simulink model "Sanepa_overall_model0x2810x29copy"  (R2022a)
settings: Solver=VariableStepAuto  StartTime=0.0  StopTime=1  RelTol=1e-3
undefined symbols (not defined in the file): D11, Delta
libraries: spsSeriesRLCLoadLib x54, spsLoadFlowBusLib x45, spsThreePhaseTransformerTwoWindingsLib x23, spsThreePhasePISectionLineLib x18, spsRMSLib x8, spsThreePhaseParallelRLCLoadLib x6, spsCurrentMeasurementLib x3, spsVoltageMeasurementLib x3, spsThreePhaseVIMeasurementLib x2, spsThreePhaseSeriesRLCBranchLib x2, spsGroundLib x1, spspowerguiLib x1
settings Model: Creator=Isha Tiwari  LastModifiedBy=neshan
settings SolverCC: AlgebraicLoopSolver=TrustRegion
settings DataIOCC: SaveOutput=off  ReturnWorkspaceOutputs=off
settings DebuggingCC: SFMachineParentedDataDiag=warning
settings ModelReferenceCC: EnableRefExpFcnMdlSchedulingChecks=off
settings RTWCC: Description=Generic Real-Time Target

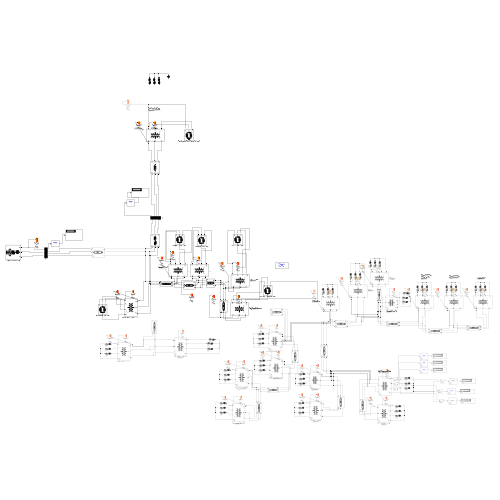
[thumbnail: Simulink's stored preview of the top-level diagram]
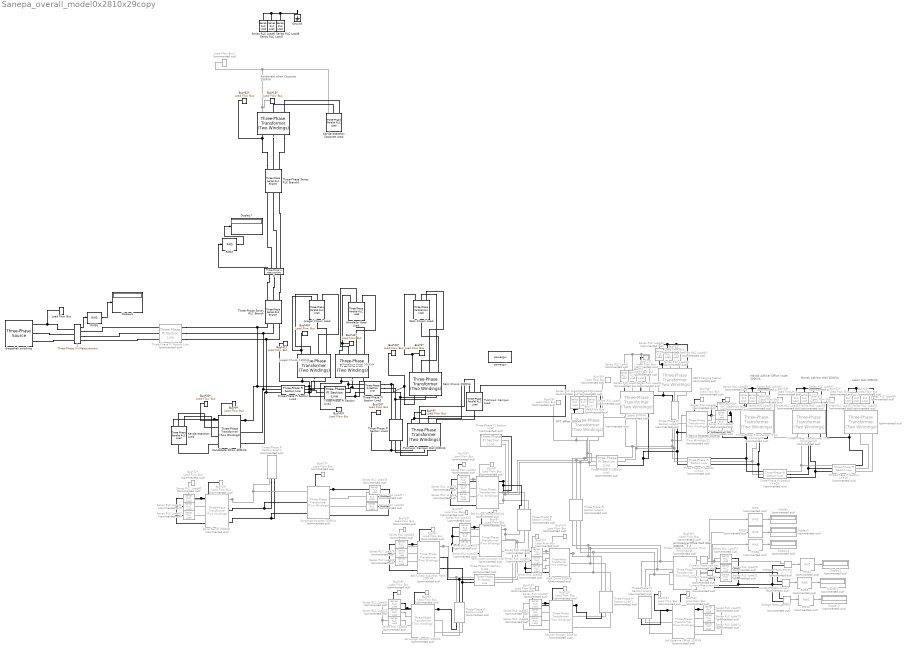
== system Sanepa_overall_model0x2810x29copy ==
  note: Norvic Hospital
      | 200KVA
  note: NTC office
      | 200KVA
  note: Manab Adhikar
      | Office inside
      | 200KVA
  note: Labim Mall
      | 200KVA
  note: Jal Utpanna Office
      | Wall Side 200KVA
  note: Manab Adhikar
      | Wall 200KVA
  note: Jwagal Chwok
      | 100KVA
  note: Himalaya Hotel
      | 300KVA
  note: Kandevata sthan
      | Opposite 250KVA
  . : spsThreePhaseTransformerTwoWindingsLib/Three-Phase Transformer (Two Windings)  Winding1Connection=Yg  Winding2Connection=Yg  CoreType=Three-limb core (core-type)  SetSaturation=off  Hysteresis=off  DataFile='hysteresis'  SetInitialFlux=off  Measurements=None  UNITS=pu  NominalPower=[ 500000 , 50 ]  Winding1=[11e3 , 0.002 , 0.08 ]  Winding2=[ 0.23e3 , 0.002 , 0.08 ]  Rm=500  Lm=500  L0=0.5  Saturation=[ 0,0 ; 0.0024,1.2 ; 1.0,1.52 ]  InitialFluxes=[ 0.8 , -0.8 , 0.7 ]  BreakLoop=off  DiscreteSolver=Trapezoidal iterative  DataType=off  TransfoNumber=1
  .. : spsThreePhaseTransformerTwoWindingsLib/Three-Phase Transformer (Two Windings)  Commented=on  Winding1Connection=Delta (D11)  Winding2Connection=Yn  CoreType=Three single-phase transformers  SetSaturation=off  Hysteresis=off  DataFile='hysteresis'  SetInitialFlux=off  Measurements=None  UNITS=pu  NominalPower=[ 200000 , 50 ]  Winding1=[ 11e3 , 0.002 , 0.08 ]  Winding2=[ 0.23e3 , 0.002 , 0.08 ]  Rm=500  Lm=500  L0=0.5  Saturation=[ 0,0 ; 0.0024,1.2 ; 1.0,1.52 ]  InitialFluxes=[ 0.8 , -0.8 , 0.7 ]  BreakLoop=off  DiscreteSolver=Trapezoidal iterative  DataType=off  TransfoNumber=1
  ... : spsThreePhaseTransformerTwoWindingsLib/Three-Phase Transformer (Two Windings)  Commented=on  Winding1Connection=Delta (D11)  Winding2Connection=Yn  CoreType=Three single-phase transformers  SetSaturation=off  Hysteresis=off  DataFile='hysteresis'  SetInitialFlux=off  Measurements=None  UNITS=pu  NominalPower=[ 200000 , 50 ]  Winding1=[11e3 , 0.002 , 0.08 ]  Winding2=[ 0.23e3 , 0.002 , 0.08 ]  Rm=500  Lm=500  L0=0.5  Saturation=[ 0,0 ; 0.0024,1.2 ; 1.0,1.52 ]  InitialFluxes=[ 0.8 , -0.8 , 0.7 ]  BreakLoop=off  DiscreteSolver=Trapezoidal iterative  DataType=off  TransfoNumber=1
  0 : spsThreePhaseVIMeasurementLib/Three-Phase V-I Measurement  VoltageMeasurement=phase-to-ground  SetLabelV=off  LabelV=V0  Vpu=on  VpuLL=off  CurrentMeasurement=no  SetLabelI=on  LabelI=I634  Ipu=off  Pbase=100e6  Vbase=11000  OutputType=Magnitude  PhasorSimulation=off  PSBequivalent=0
  1 : spsThreePhaseVIMeasurementLib/Three-Phase V-I Measurement  VoltageMeasurement=phase-to-ground  SetLabelV=off  LabelV=V0  Vpu=on  VpuLL=off  CurrentMeasurement=no  SetLabelI=on  LabelI=I634  Ipu=off  Pbase=100e6  Vbase=11000  OutputType=Magnitude  PhasorSimulation=off  PSBequivalent=0
  Bakhundol Carwash 200KVA : spsThreePhaseTransformerTwoWindingsLib/Three-Phase Transformer (Two Windings)  Commented=on  Winding1Connection=Delta (D11)  Winding2Connection=Yn  CoreType=Three single-phase transformers  SetSaturation=off  Hysteresis=off  DataFile='hysteresis'  SetInitialFlux=off  Measurements=None  UNITS=pu  NominalPower=[ 200000 , 50 ]  Winding1=[ 11e3 , 0.002 , 0.08 ]  Winding2=[ 0.23e3 , 0.002 , 0.08 ]  Rm=500  Lm=500  L0=0.5  Saturation=[ 0,0 ; 0.0024,1.2 ; 1.0,1.52 ]  InitialFluxes=[ 0.8 , -0.8 , 0.7 ]  BreakLoop=off  DiscreteSolver=Trapezoidal iterative  DataType=off  TransfoNumber=1
  Bakhundol Kutumba Hotel 200KVA : spsThreePhaseTransformerTwoWindingsLib/Three-Phase Transformer (Two Windings)  Commented=on  Winding1Connection=Delta (D11)  Winding2Connection=Yn  CoreType=Three single-phase transformers  SetSaturation=off  Hysteresis=off  DataFile='hysteresis'  SetInitialFlux=off  Measurements=None  UNITS=pu  NominalPower=[ 200000 , 50 ]  Winding1=[ 11e3 , 0.002 , 0.08 ]  Winding2=[ 0.23e3 , 0.002 , 0.08 ]  Rm=500  Lm=500  L0=0.5  Saturation=[ 0,0 ; 0.0024,1.2 ; 1.0,1.52 ]  InitialFluxes=[ 0.8 , -0.8 , 0.7 ]  BreakLoop=off  DiscreteSolver=Trapezoidal iterative  DataType=off  TransfoNumber=1
  Bakhundol Mode 300KVA : spsThreePhaseTransformerTwoWindingsLib/Three-Phase Transformer (Two Windings)  Commented=on  Winding1Connection=Delta (D11)  Winding2Connection=Yn  CoreType=Three single-phase transformers  SetSaturation=off  Hysteresis=off  DataFile='hysteresis'  SetInitialFlux=off  Measurements=None  UNITS=pu  NominalPower=[ 300000 , 50 ]  Winding1=[ 11e3 , 0.002 , 0.08 ]  Winding2=[ 0.23e3 , 0.002 , 0.08 ]  Rm=500  Lm=500  L0=0.5  Saturation=[ 0,0 ; 0.0024,1.2 ; 1.0,1.52 ]  InitialFluxes=[ 0.8 , -0.8 , 0.7 ]  BreakLoop=off  DiscreteSolver=Trapezoidal iterative  DataType=off  TransfoNumber=1
  Bima Samiti 200KVA : spsThreePhaseTransformerTwoWindingsLib/Three-Phase Transformer (Two Windings)  Commented=on  Winding1Connection=Delta (D11)  Winding2Connection=Yn  CoreType=Three single-phase transformers  SetSaturation=off  Hysteresis=off  DataFile='hysteresis'  SetInitialFlux=off  Measurements=None  UNITS=pu  NominalPower=[ 200000 , 50 ]  Winding1=[ 11e3 , 0.002 , 0.08 ]  Winding2=[ 0.23e3 , 0.002 , 0.08 ]  Rm=500  Lm=500  L0=0.5  Saturation=[ 0,0 ; 0.0024,1.2 ; 1.0,1.52 ]  InitialFluxes=[ 0.8 , -0.8 , 0.7 ]  BreakLoop=off  DiscreteSolver=Trapezoidal iterative  DataType=off  TransfoNumber=1
  Bus*1* : spsLoadFlowBusLib/Load Flow Bus  Commented=on  LConnTagsString=a  Phases=single  Connectors=on one side  ID=Bus*1*  Vbase=400  Vref=1  Vangle=0  VLF=1  VLFb=1  VLFc=1  angleLF=0  angleLFb=0  angleLFc=0
      settings: SourceProductBaseCode=PS
  Bus*10* : spsLoadFlowBusLib/Load Flow Bus  Commented=on  LConnTagsString=a  Phases=single  Connectors=on one side  ID=Bus*10*  Vbase=230  Vref=1  Vangle=0  VLF=1  VLFb=1  VLFc=1  angleLF=0  angleLFb=0  angleLFc=0
      settings: SourceProductBaseCode=PS
  Bus*11* : spsLoadFlowBusLib/Load Flow Bus  Commented=on  LConnTagsString=a  Phases=single  Connectors=on one side  ID=Bus*11*  Vbase=230  Vref=1  Vangle=0  VLF=1  VLFb=1  VLFc=1  angleLF=0  angleLFb=0  angleLFc=0
      settings: SourceProductBaseCode=PS
  Bus*12* : spsLoadFlowBusLib/Load Flow Bus  Commented=on  LConnTagsString=a  Phases=single  Connectors=on one side  ID=Bus*12*  Vbase=230  Vref=1  Vangle=0  VLF=1  VLFb=1  VLFc=1  angleLF=0  angleLFb=0  angleLFc=0
      settings: SourceProductBaseCode=PS
  Bus*13* : spsLoadFlowBusLib/Load Flow Bus  LConnTagsString=a  Phases=single  Connectors=on one side  ID=Bus*13*  Vbase=230  Vref=1  Vangle=0  VLF=0.9989  VLFb=1  VLFc=1  angleLF=-0.1488  angleLFb=0  angleLFc=0
      settings: SourceProductBaseCode=PS
  Bus*14* : spsLoadFlowBusLib/Load Flow Bus  Commented=on  LConnTagsString=a  Phases=single  Connectors=on one side  ID=Bus*14*  Vbase=230  Vref=1  Vangle=0  VLF=1  VLFb=1  VLFc=1  angleLF=0  angleLFb=0  angleLFc=0
      settings: SourceProductBaseCode=PS
  Bus*15* : spsLoadFlowBusLib/Load Flow Bus  Commented=on  LConnTagsString=a  Phases=single  Connectors=on one side  ID=Bus*15*  Vbase=230  Vref=1  Vangle=0  VLF=1  VLFb=1  VLFc=1  angleLF=0  angleLFb=0  angleLFc=0
      settings: SourceProductBaseCode=PS
  Bus*16* : spsLoadFlowBusLib/Load Flow Bus  Commented=on  LConnTagsString=a  Phases=single  Connectors=on one side  ID=Bus*16*  Vbase=230  Vref=1  Vangle=0  VLF=1  VLFb=1  VLFc=1  angleLF=0  angleLFb=0  angleLFc=0
      settings: SourceProductBaseCode=PS
  Bus*17* : spsLoadFlowBusLib/Load Flow Bus  Commented=on  LConnTagsString=a  Phases=single  Connectors=on one side  ID=Bus*17*  Vbase=230  Vref=1  Vangle=0  VLF=1  VLFb=1  VLFc=1  angleLF=0  angleLFb=0  angleLFc=0
      settings: SourceProductBaseCode=PS
  Bus*18* : spsLoadFlowBusLib/Load Flow Bus  Commented=on  LConnTagsString=a  Phases=single  Connectors=on one side  ID=Bus*18*  Vbase=11000  Vref=1  Vangle=0  VLF=1  VLFb=1  VLFc=1  angleLF=0  angleLFb=0  angleLFc=0
      settings: SourceProductBaseCode=PS
  Bus*19* : spsLoadFlowBusLib/Load Flow Bus  Commented=on  LConnTagsString=a  Phases=single  Connectors=on one side  ID=Bus*19*  Vbase=11000  Vref=1  Vangle=0  VLF=1  VLFb=1  VLFc=1  angleLF=0  angleLFb=0  angleLFc=0
      settings: SourceProductBaseCode=PS
  Bus*2* : spsLoadFlowBusLib/Load Flow Bus  LConnTagsString=a  Phases=single  Connectors=on one side  ID=Bus*2*  Vbase=230  Vref=1  Vangle=0  VLF=1  VLFb=1  VLFc=1  angleLF=0  angleLFb=0  angleLFc=0
      settings: SourceProductBaseCode=PS
  Bus*20* : spsLoadFlowBusLib/Load Flow Bus  Commented=on  LConnTagsString=a  Phases=single  Connectors=on one side  ID=Bus*20*  Vbase=11000  Vref=1  Vangle=0  VLF=1  VLFb=1  VLFc=1  angleLF=0  angleLFb=0  angleLFc=0
      settings: SourceProductBaseCode=PS
  Bus*21* : spsLoadFlowBusLib/Load Flow Bus  Commented=on  LConnTagsString=a  Phases=single  Connectors=on one side  ID=Bus*21*  Vbase=11000  Vref=1  Vangle=0  VLF=1  VLFb=1  VLFc=1  angleLF=0  angleLFb=0  angleLFc=0
      settings: SourceProductBaseCode=PS
  Bus*22* : spsLoadFlowBusLib/Load Flow Bus  Commented=on  LConnTagsString=a  Phases=single  Connectors=on one side  ID=Bus*22*  Vbase=11000  Vref=1  Vangle=0  VLF=1  VLFb=1  VLFc=1  angleLF=0  angleLFb=0  angleLFc=0
      settings: SourceProductBaseCode=PS
  Bus*23* : spsLoadFlowBusLib/Load Flow Bus  LConnTagsString=a  Phases=single  Connectors=on one side  ID=Bus*23*  Vbase=11000  Vref=1  Vangle=0  VLF=1  VLFb=1  VLFc=1  angleLF=0  angleLFb=0  angleLFc=0
      settings: SourceProductBaseCode=PS
  Bus*24* : spsLoadFlowBusLib/Load Flow Bus  Commented=on  LConnTagsString=a  Phases=single  Connectors=on one side  ID=Bus*24*  Vbase=11000  Vref=1  Vangle=0  VLF=1  VLFb=1  VLFc=1  angleLF=0  angleLFb=0  angleLFc=0
      settings: SourceProductBaseCode=PS
  Bus*25* : spsLoadFlowBusLib/Load Flow Bus  Commented=on  LConnTagsString=a  Phases=single  Connectors=on one side  ID=Bus*25*  Vbase=11000  Vref=1  Vangle=0  VLF=1  VLFb=1  VLFc=1  angleLF=0  angleLFb=0  angleLFc=0
      settings: SourceProductBaseCode=PS
  Bus*26* : spsLoadFlowBusLib/Load Flow Bus  LConnTagsString=a  Phases=single  Connectors=on one side  ID=Bus*26*  Vbase=11000  Vref=1  Vangle=0  VLF=1  VLFb=1  VLFc=1  angleLF=0  angleLFb=0  angleLFc=0
      settings: SourceProductBaseCode=PS
  Bus*27* : spsLoadFlowBusLib/Load Flow Bus  Commented=on  LConnTagsString=a  Phases=single  Connectors=on one side  ID=Bus*27*  Vbase=11000  Vref=1  Vangle=0  VLF=1  VLFb=1  VLFc=1  angleLF=0  angleLFb=0  angleLFc=0
      settings: SourceProductBaseCode=PS
  Bus*28* : spsLoadFlowBusLib/Load Flow Bus  Commented=on  LConnTagsString=a  Phases=single  Connectors=on one side  ID=Bus*28*  Vbase=11000  Vref=1  Vangle=0  VLF=1  VLFb=1  VLFc=1  angleLF=0  angleLFb=0  angleLFc=0
      settings: SourceProductBaseCode=PS
  Bus*29* : spsLoadFlowBusLib/Load Flow Bus  Commented=on  LConnTagsString=a  Phases=single  Connectors=on one side  ID=Bus*29*  Vbase=11000  Vref=1  Vangle=0  VLF=1  VLFb=1  VLFc=1  angleLF=0  angleLFb=0  angleLFc=0
      settings: SourceProductBaseCode=PS
  Bus*3* : spsLoadFlowBusLib/Load Flow Bus  LConnTagsString=a  Phases=single  Connectors=on one side  ID=Bus*3*  Vbase=230  Vref=1  Vangle=0  VLF=1  VLFb=1  VLFc=1  angleLF=0  angleLFb=0  angleLFc=0
      settings: SourceProductBaseCode=PS
  Bus*30* : spsLoadFlowBusLib/Load Flow Bus  LConnTagsString=a  Phases=single  Connectors=on one side  ID=Bus*30*  Vbase=11000  Vref=1  Vangle=0  VLF=1  VLFb=1  VLFc=1  angleLF=0  angleLFb=0  angleLFc=0
      settings: SourceProductBaseCode=PS
  Bus*31* : spsLoadFlowBusLib/Load Flow Bus  LConnTagsString=a  Phases=single  Connectors=on one side  ID=Bus*31*  Vbase=11000  Vref=1  Vangle=0  VLF=0.9999  VLFb=1  VLFc=1  angleLF=-0.004876  angleLFb=0  angleLFc=0
      settings: SourceProductBaseCode=PS
  Bus*32* : spsLoadFlowBusLib/Load Flow Bus  Commented=on  LConnTagsString=a  Phases=single  Connectors=on one side  ID=Bus*32*  Vbase=230  Vref=1  Vangle=0  VLF=1  VLFb=1  VLFc=1  angleLF=0  angleLFb=0  angleLFc=0
      settings: SourceProductBaseCode=PS
  Bus*33* : spsLoadFlowBusLib/Load Flow Bus  Commented=on  LConnTagsString=a  Phases=single  Connectors=on one side  ID=Bus*33*  Vbase=11000  Vref=1  Vangle=0  VLF=1  VLFb=1  VLFc=1  angleLF=0  angleLFb=0  angleLFc=0
      settings: SourceProductBaseCode=PS
  Bus*34* : spsLoadFlowBusLib/Load Flow Bus  Commented=on  LConnTagsString=a  Phases=single  Connectors=on one side  ID=Bus*34*  Vbase=230  Vref=1  Vangle=0  VLF=1  VLFb=1  VLFc=1  angleLF=0  angleLFb=0  angleLFc=0
      settings: SourceProductBaseCode=PS
  Bus*35* : spsLoadFlowBusLib/Load Flow Bus  Commented=on  LConnTagsString=a  Phases=single  Connectors=on one side  ID=Bus*35*  Vbase=11000  Vref=1  Vangle=0  VLF=1  VLFb=1  VLFc=1  angleLF=0  angleLFb=0  angleLFc=0
      settings: SourceProductBaseCode=PS
  Bus*36* : spsLoadFlowBusLib/Load Flow Bus  Commented=on  LConnTagsString=a  Phases=single  Connectors=on one side  ID=Bus*36*  Vbase=230  Vref=1  Vangle=0  VLF=1  VLFb=1  VLFc=1  angleLF=0  angleLFb=0  angleLFc=0
      settings: SourceProductBaseCode=PS
  Bus*37* : spsLoadFlowBusLib/Load Flow Bus  Commented=on  LConnTagsString=a  Phases=single  Connectors=on one side  ID=Bus*37*  Vbase=11000  Vref=1  Vangle=0  VLF=1  VLFb=1  VLFc=1  angleLF=0  angleLFb=0  angleLFc=0
      settings: SourceProductBaseCode=PS
  Bus*38* : spsLoadFlowBusLib/Load Flow Bus  Commented=on  LConnTagsString=a  Phases=single  Connectors=on one side  ID=Bus*38*  Vbase=230  Vref=1  Vangle=0  VLF=1  VLFb=1  VLFc=1  angleLF=0  angleLFb=0  angleLFc=0
      settings: SourceProductBaseCode=PS
  Bus*39* : spsLoadFlowBusLib/Load Flow Bus  Commented=on  LConnTagsString=a  Phases=single  Connectors=on one side  ID=Bus*39*  Vbase=11000  Vref=1  Vangle=0  VLF=1  VLFb=1  VLFc=1  angleLF=0  angleLFb=0  angleLFc=0
      settings: SourceProductBaseCode=PS
  Bus*4* : spsLoadFlowBusLib/Load Flow Bus  Commented=on  LConnTagsString=a  Phases=single  Connectors=on one side  ID=Bus*4*  Vbase=230  Vref=1  Vangle=0  VLF=1  VLFb=1  VLFc=1  angleLF=0  angleLFb=0  angleLFc=0
      settings: SourceProductBaseCode=PS
  Bus*40* : spsLoadFlowBusLib/Load Flow Bus  LConnTagsString=a  Phases=single  Connectors=on one side  ID=Bus*40*  Vbase=230  Vref=1  Vangle=0  VLF=1  VLFb=1  VLFc=1  angleLF=0  angleLFb=0  angleLFc=0
      settings: SourceProductBaseCode=PS
  Bus*41* : spsLoadFlowBusLib/Load Flow Bus  LConnTagsString=a  Phases=single  Connectors=on one side  ID=Bus*41*  Vbase=11000  Vref=1  Vangle=0  VLF=1  VLFb=1  VLFc=1  angleLF=0  angleLFb=0  angleLFc=0
      settings: SourceProductBaseCode=PS
  Bus*42* : spsLoadFlowBusLib/Load Flow Bus  LConnTagsString=a  Phases=single  Connectors=on one side  ID=Bus*42*  Vbase=230  Vref=1  Vangle=0  VLF=1  VLFb=1  VLFc=1  angleLF=0  angleLFb=0  angleLFc=0
      settings: SourceProductBaseCode=PS
  Bus*43* : spsLoadFlowBusLib/Load Flow Bus  LConnTagsString=a  Phases=single  Connectors=on one side  ID=Bus*43*  Vbase=11000  Vref=1  Vangle=0  VLF=1  VLFb=1  VLFc=1  angleLF=0  angleLFb=0  angleLFc=0
      settings: SourceProductBaseCode=PS
  Bus*5* : spsLoadFlowBusLib/Load Flow Bus  Commented=on  LConnTagsString=a  Phases=single  Connectors=on one side  ID=Bus*5*  Vbase=230  Vref=1  Vangle=0  VLF=1  VLFb=1  VLFc=1  angleLF=0  angleLFb=0  angleLFc=0
      settings: SourceProductBaseCode=PS
  Bus*6* : spsLoadFlowBusLib/Load Flow Bus  Commented=on  LConnTagsString=a  Phases=single  Connectors=on one side  ID=Bus*6*  Vbase=230  Vref=1  Vangle=0  VLF=1  VLFb=1  VLFc=1  angleLF=0  angleLFb=0  angleLFc=0
      settings: SourceProductBaseCode=PS
  Bus*7* : spsLoadFlowBusLib/Load Flow Bus  Commented=on  LConnTagsString=a  Phases=single  Connectors=on one side  ID=Bus*7*  Vbase=230  Vref=1  Vangle=0  VLF=1  VLFb=1  VLFc=1  angleLF=0  angleLFb=0  angleLFc=0
      settings: SourceProductBaseCode=PS
  Bus*8* : spsLoadFlowBusLib/Load Flow Bus  Commented=on  LConnTagsString=a  Phases=single  Connectors=on one side  ID=Bus*8*  Vbase=230  Vref=1  Vangle=0  VLF=1  VLFb=1  VLFc=1  angleLF=0  angleLFb=0  angleLFc=0
      settings: SourceProductBaseCode=PS
  Bus*9* : spsLoadFlowBusLib/Load Flow Bus  LConnTagsString=a  Phases=single  Connectors=on one side  ID=Bus*9*  Vbase=230  Vref=1  Vangle=0  VLF=1  VLFb=1  VLFc=1  angleLF=0  angleLFb=0  angleLFc=0
      settings: SourceProductBaseCode=PS
  Current Measurement : spsCurrentMeasurementLib/Current Measurement  Commented=on  PhasorSimulation=off  OutputType=Complex  PSBequivalent=0
  Current Measurement3 : spsCurrentMeasurementLib/Current Measurement  Commented=on  PhasorSimulation=off  OutputType=Complex  PSBequivalent=0
  Current Measurement4 : spsCurrentMeasurementLib/Current Measurement  Commented=on  PhasorSimulation=off  OutputType=Complex  PSBequivalent=0
  Display{,1..5} (6 alike) : Display  Commented=on
  Display6 : Display
  Display7 : Display
  Ground : spsGroundLib/Ground  LConnTagsString=a
  HImalaya Hotel Load : spsThreePhaseParallelRLCLoadLib/Three-Phase Parallel RLC Load  LConnTagsString=A|B|C  RConnTagsString=N  Configuration=Y (neutral)  NominalVoltage=230  Vabc=[1e3 1e3 1e3]  Vabcp=[1e3 1e3 1e3]  NominalFrequency=50  UnbalancedPower=off  ActivePower=29497.5  InductivePower=9695.359  CapacitivePower=0  Pabc=[22287 23379.5 18572.5]  QLabc=[7325.383 7684.47 6104.48]  QCabc=[0 0 0]  Pabcp=[10e3 9e3 11e3]  QLabcp=[100 90 110]  QCabcp=[100 90 110]  Measurements=None  LoadType=constant PQ
  High Court 200KVA : spsThreePhaseTransformerTwoWindingsLib/Three-Phase Transformer (Two Windings)  Commented=on  Winding1Connection=Delta (D11)  Winding2Connection=Yn  CoreType=Three single-phase transformers  SetSaturation=off  Hysteresis=off  DataFile='hysteresis'  SetInitialFlux=off  Measurements=None  UNITS=pu  NominalPower=[ 200000 , 50 ]  Winding1=[ 11e3 , 0.002 , 0.08 ]  Winding2=[ 0.23e3 , 0.002 , 0.08 ]  Rm=500  Lm=500  L0=0.5  Saturation=[ 0,0 ; 0.0024,1.2 ; 1.0,1.52 ]  InitialFluxes=[ 0.8 , -0.8 , 0.7 ]  BreakLoop=off  DiscreteSolver=Trapezoidal iterative  DataType=off  TransfoNumber=1
  Jall Utpanna Office 100KVA : spsThreePhaseTransformerTwoWindingsLib/Three-Phase Transformer (Two Windings)  Commented=on  Winding1Connection=Delta (D11)  Winding2Connection=Yn  CoreType=Three single-phase transformers  SetSaturation=off  Hysteresis=off  DataFile='hysteresis'  SetInitialFlux=off  Measurements=None  UNITS=pu  NominalPower=[ 100000 , 50 ]  Winding1=[ 11e3 , 0.002 , 0.08 ]  Winding2=[ 0.23e3 , 0.002 , 0.08 ]  Rm=500  Lm=500  L0=0.5  Saturation=[ 0,0 ; 0.0024,1.2 ; 1.0,1.52 ]  InitialFluxes=[ 0.8 , -0.8 , 0.7 ]  BreakLoop=off  DiscreteSolver=Trapezoidal iterative  DataType=off  TransfoNumber=1
  Jwagal Chowk Load : spsThreePhaseParallelRLCLoadLib/Three-Phase Parallel RLC Load  LConnTagsString=A|B|C  RConnTagsString=N  Configuration=Y (neutral)  NominalVoltage=230  Vabc=[1e3 1e3 1e3]  Vabcp=[1e3 1e3 1e3]  NominalFrequency=50  UnbalancedPower=off  ActivePower=21850  InductivePower=7181.748  CapacitivePower=0  Pabc=[22287 23379.5 18572.5]  QLabc=[7325.383 7684.47 6104.48]  QCabc=[0 0 0]  Pabcp=[10e3 9e3 11e3]  QLabcp=[100 90 110]  QCabcp=[100 90 110]  Measurements=None  LoadType=constant PQ
  Kandebata Sthan 300KVA : spsThreePhaseTransformerTwoWindingsLib/Three-Phase Transformer (Two Windings)  Winding1Connection=Delta (D11)  Winding2Connection=Yn  CoreType=Three single-phase transformers  SetSaturation=off  Hysteresis=off  DataFile='hysteresis'  SetInitialFlux=off  Measurements=None  UNITS=pu  NominalPower=[ 300000 , 50 ]  Winding1=[ 11e3 , 0.002 , 0.08 ]  Winding2=[ 0.23e3 , 0.002 , 0.08 ]  Rm=500  Lm=500  L0=0.5  Saturation=[ 0,0 ; 0.0024,1.2 ; 1.0,1.52 ]  InitialFluxes=[ 0.8 , -0.8 , 0.7 ]  BreakLoop=off  DiscreteSolver=Trapezoidal iterative  DataType=off  TransfoNumber=1
  Kandevatasthan Load : spsThreePhaseParallelRLCLoadLib/Three-Phase Parallel RLC Load  LConnTagsString=A|B|C  RConnTagsString=N  Configuration=Y (neutral)  NominalVoltage=230  Vabc=[1e3 1e3 1e3]  Vabcp=[1e3 1e3 1e3]  NominalFrequency=50  UnbalancedPower=off  ActivePower=68827.5  InductivePower=22622.506  CapacitivePower=0  Pabc=[22287 23379.5 18572.5]  QLabc=[7325.383 7684.47 6104.48]  QCabc=[0 0 0]  Pabcp=[10e3 9e3 11e3]  QLabcp=[100 90 110]  QCabcp=[100 90 110]  Measurements=None  LoadType=constant PQ
  Kandevatasthan Opposite Load : spsThreePhaseParallelRLCLoadLib/Three-Phase Parallel RLC Load  LConnTagsString=A|B|C  Configuration=Y (grounded)  NominalVoltage=230  Vabc=[1e3 1e3 1e3]  Vabcp=[1e3 1e3 1e3]  NominalFrequency=50  UnbalancedPower=off  ActivePower=64239  InductivePower=21114.33  CapacitivePower=0  Pabc=[22287 23379.5 18572.5]  QLabc=[7325.383 7684.47 6104.48]  QCabc=[0 0 0]  Pabcp=[10e3 9e3 11e3]  QLabcp=[100 90 110]  QCabcp=[100 90 110]  Measurements=None  LoadType=constant PQ
  Load Flow Bus : spsLoadFlowBusLib/Load Flow Bus  LConnTagsString=a  Phases=single  Connectors=on one side  ID=BUS_1  Vbase=11e3  Vref=1  Vangle=0  VLF=1  VLFb=1  VLFc=1  angleLF=0  angleLFb=0  angleLFc=0
      settings: SourceProductBaseCode=PS
  Load Flow Bus1 : spsLoadFlowBusLib/Load Flow Bus  Commented=on  LConnTagsString=a  Phases=single  Connectors=on one side  ID=BUS_2  Vbase=11e3  Vref=1  Vangle=0  VLF=1  VLFb=1  VLFc=1  angleLF=0  angleLFb=0  angleLFc=0
      settings: SourceProductBaseCode=PS
  NEA Charging Station : spsThreePhaseTransformerTwoWindingsLib/Three-Phase Transformer (Two Windings)  Commented=on  Winding1Connection=Delta (D11)  Winding2Connection=Yn  CoreType=Three single-phase transformers  SetSaturation=off  Hysteresis=off  DataFile='hysteresis'  SetInitialFlux=off  Measurements=None  UNITS=pu  NominalPower=[ 200000 , 50 ]  Winding1=[ 11e3 , 0.002 , 0.08 ]  Winding2=[ 0.23e3 , 0.002 , 0.08 ]  Rm=500  Lm=500  L0=0.5  Saturation=[ 0,0 ; 0.0024,1.2 ; 1.0,1.52 ]  InitialFluxes=[ 0.8 , -0.8 , 0.7 ]  BreakLoop=off  DiscreteSolver=Trapezoidal iterative  DataType=off  TransfoNumber=1
  Pariwar Niyojan 100KVA : spsThreePhaseTransformerTwoWindingsLib/Three-Phase Transformer (Two Windings)  Commented=on  Winding1Connection=Delta (D11)  Winding2Connection=Yn  CoreType=Three single-phase transformers  SetSaturation=off  Hysteresis=off  DataFile='hysteresis'  SetInitialFlux=off  Measurements=None  UNITS=pu  NominalPower=[ 100000 , 50 ]  Winding1=[ 11e3 , 0.002 , 0.08 ]  Winding2=[ 0.23e3 , 0.002 , 0.08 ]  Rm=500  Lm=500  L0=0.5  Saturation=[ 0,0 ; 0.0024,1.2 ; 1.0,1.52 ]  InitialFluxes=[ 0.8 , -0.8 , 0.7 ]  BreakLoop=off  DiscreteSolver=Trapezoidal iterative  DataType=off  TransfoNumber=1
  Pulchowk Campus Load : spsThreePhaseParallelRLCLoadLib/Three-Phase Parallel RLC Load  LConnTagsString=A|B|C  RConnTagsString=N  Configuration=Y (neutral)  NominalVoltage=230  Vabc=[1e3 1e3 1e3]  Vabcp=[1e3 1e3 1e3]  NominalFrequency=50  UnbalancedPower=off  ActivePower=38019.33  InductivePower=12496.241  CapacitivePower=0  Pabc=[22287 23379.5 18572.5]  QLabc=[7325.383 7684.47 6104.48]  QCabc=[0 0 0]  Pabcp=[10e3 9e3 11e3]  QLabcp=[100 90 110]  QCabcp=[100 90 110]  Measurements=None  LoadType=constant PQ
  Pulchwok Campus Wall 200KVA : spsThreePhaseTransformerTwoWindingsLib/Three-Phase Transformer (Two Windings)  Winding1Connection=Delta (D11)  Winding2Connection=Yn  CoreType=Three single-phase transformers  SetSaturation=off  Hysteresis=off  DataFile='hysteresis'  SetInitialFlux=off  Measurements=None  UNITS=pu  NominalPower=[ 100000 , 50 ]  Winding1=[ 11e3 , 0.002 , 0.08 ]  Winding2=[ 0.23e3 , 0.002 , 0.08 ]  Rm=500  Lm=500  L0=0.5  Saturation=[ 0,0 ; 0.0024,1.2 ; 1.0,1.52 ]  InitialFluxes=[ 0.8 , -0.8 , 0.7 ]  BreakLoop=off  DiscreteSolver=Trapezoidal iterative  DataType=off  TransfoNumber=1
  RMS{,1..5} (6 alike) : spsRMSLib/RMS  Commented=on  TrueRMS=on  Freq=50  RMSInit=0  Ts=0
  RMS6 : spsRMSLib/RMS  TrueRMS=on  Freq=60  RMSInit=120  Ts=0
  RMS7 : spsRMSLib/RMS  TrueRMS=on  Freq=60  RMSInit=0  Ts=0
  Sajha 500KVA : spsThreePhaseTransformerTwoWindingsLib/Three-Phase Transformer (Two Windings)  Commented=on  Winding1Connection=Delta (D11)  Winding2Connection=Yn  CoreType=Three single-phase transformers  SetSaturation=off  Hysteresis=off  DataFile='hysteresis'  SetInitialFlux=off  Measurements=None  UNITS=pu  NominalPower=[ 500000 , 50 ]  Winding1=[ 11e3 , 0.002 , 0.08 ]  Winding2=[ 0.40e3 , 0.002 , 0.08 ]  Rm=500  Lm=500  L0=0.5  Saturation=[ 0,0 ; 0.0024,1.2 ; 1.0,1.52 ]  InitialFluxes=[ 0.8 , -0.8 , 0.7 ]  BreakLoop=off  DiscreteSolver=Trapezoidal iterative  DataType=off  TransfoNumber=1
  Salik Chowk Load : spsThreePhaseParallelRLCLoadLib/Three-Phase Parallel RLC Load  LConnTagsString=A|B|C  RConnTagsString=N  Configuration=Y (neutral)  NominalVoltage=230  Vabc=[1e3 1e3 1e3]  Vabcp=[1e3 1e3 1e3]  NominalFrequency=50  UnbalancedPower=off  ActivePower=19883.5  InductivePower=6535.388  CapacitivePower=0  Pabc=[22287 23379.5 18572.5]  QLabc=[7325.383 7684.47 6104.48]  QCabc=[0 0 0]  Pabcp=[10e3 9e3 11e3]  QLabcp=[100 90 110]  QCabcp=[100 90 110]  Measurements=None  LoadType=constant PQ
  Salik Chwok 200KVA : spsThreePhaseTransformerTwoWindingsLib/Three-Phase Transformer (Two Windings)  Winding1Connection=Delta (D11)  Winding2Connection=Yn  CoreType=Three single-phase transformers  SetSaturation=off  Hysteresis=off  DataFile='hysteresis'  SetInitialFlux=off  Measurements=None  UNITS=pu  NominalPower=[ 200000 , 50 ]  Winding1=[11e3 , 0.002 , 0.08 ]  Winding2=[ 0.23e3 , 0.002 , 0.08 ]  Rm=500  Lm=500  L0=0.5  Saturation=[ 0,0 ; 0.0024,1.2 ; 1.0,1.52 ]  InitialFluxes=[ 0.8 , -0.8 , 0.7 ]  BreakLoop=off  DiscreteSolver=Trapezoidal iterative  DataType=off  TransfoNumber=1
  Sarbanga Hospital 200KVA : spsThreePhaseTransformerTwoWindingsLib/Three-Phase Transformer (Two Windings)  Commented=on  Winding1Connection=Delta (D11)  Winding2Connection=Yn  CoreType=Three single-phase transformers  SetSaturation=off  Hysteresis=off  DataFile='hysteresis'  SetInitialFlux=off  Measurements=None  UNITS=pu  NominalPower=[ 200000 , 50 ]  Winding1=[ 11e3 , 0.002 , 0.08 ]  Winding2=[ 0.23e3 , 0.002 , 0.08 ]  Rm=500  Lm=500  L0=0.5  Saturation=[ 0,0 ; 0.0024,1.2 ; 1.0,1.52 ]  InitialFluxes=[ 0.8 , -0.8 , 0.7 ]  BreakLoop=off  DiscreteSolver=Trapezoidal iterative  DataType=off  TransfoNumber=1
  Sarwanga Hospital 300KVA : spsThreePhaseTransformerTwoWindingsLib/Three-Phase Transformer (Two Windings)  Commented=on  Winding1Connection=Delta (D11)  Winding2Connection=Yn  CoreType=Three single-phase transformers  SetSaturation=off  Hysteresis=off  DataFile='hysteresis'  SetInitialFlux=off  Measurements=None  UNITS=pu  NominalPower=[ 300000 , 50 ]  Winding1=[ 11e3 , 0.002 , 0.08 ]  Winding2=[ 0.23e3 , 0.002 , 0.08 ]  Rm=500  Lm=500  L0=0.5  Saturation=[ 0,0 ; 0.0024,1.2 ; 1.0,1.52 ]  InitialFluxes=[ 0.8 , -0.8 , 0.7 ]  BreakLoop=off  DiscreteSolver=Trapezoidal iterative  DataType=off  TransfoNumber=1
  Series RLC Load1 : spsSeriesRLCLoadLib/Series RLC Load  Commented=on  LConnTagsString=a  RConnTagsString=__new0  NominalVoltage=230  NominalFrequency=50  ActivePower=50255  InductivePower=16518.02  CapacitivePower=0  Setx0=off  InitialVoltage=0  SetiL0=off  InitialCurrent=0  Measurements=None  LoadType=constant Z
  Series RLC Load2 : spsSeriesRLCLoadLib/Series RLC Load  Commented=on  LConnTagsString=a  RConnTagsString=__new0  NominalVoltage=230  NominalFrequency=50  ActivePower=32775  InductivePower=10772.62  CapacitivePower=0  Setx0=off  InitialVoltage=0  SetiL0=off  InitialCurrent=0  Measurements=None  LoadType=constant Z
  Series RLC Load21 : spsSeriesRLCLoadLib/Series RLC Load  Commented=on  LConnTagsString=a  RConnTagsString=__new0  NominalVoltage=230  NominalFrequency=50  ActivePower=21850  InductivePower=7181.75  CapacitivePower=0  Setx0=off  InitialVoltage=0  SetiL0=off  InitialCurrent=0  Measurements=None  LoadType=constant Z
  Series RLC Load22 : spsSeriesRLCLoadLib/Series RLC Load  Commented=on  LConnTagsString=a  RConnTagsString=__new0  NominalVoltage=230  NominalFrequency=50  ActivePower=19665  InductivePower=6463.573  CapacitivePower=0  Setx0=off  InitialVoltage=0  SetiL0=off  InitialCurrent=0  Measurements=None  LoadType=constant Z
  Series RLC Load23 : spsSeriesRLCLoadLib/Series RLC Load  Commented=on  LConnTagsString=a  RConnTagsString=__new0  NominalVoltage=230  NominalFrequency=50  ActivePower=19446.5  InductivePower=6391.755  CapacitivePower=0  Setx0=off  InitialVoltage=0  SetiL0=off  InitialCurrent=0  Measurements=None  LoadType=constant Z
  Series RLC Load24 : spsSeriesRLCLoadLib/Series RLC Load  Commented=on  LConnTagsString=a  RConnTagsString=__new0  NominalVoltage=230  NominalFrequency=50  ActivePower=20539  InductivePower=6750.843  CapacitivePower=0  Setx0=off  InitialVoltage=0  SetiL0=off  InitialCurrent=0  Measurements=None  LoadType=constant Z
  Series RLC Load25 : spsSeriesRLCLoadLib/Series RLC Load  Commented=on  LConnTagsString=a  RConnTagsString=__new0  NominalVoltage=230  NominalFrequency=50  ActivePower=7647.5  InductivePower=2513.612  CapacitivePower=0  Setx0=off  InitialVoltage=0  SetiL0=off  InitialCurrent=0  Measurements=None  LoadType=constant Z
  Series RLC Load26 : spsSeriesRLCLoadLib/Series RLC Load  Commented=on  LConnTagsString=a  RConnTagsString=__new0  NominalVoltage=230  NominalFrequency=50  ActivePower=1529.5  InductivePower=502.72  CapacitivePower=0  Setx0=off  InitialVoltage=0  SetiL0=off  InitialCurrent=0  Measurements=None  LoadType=constant Z
  Series RLC Load27 : spsSeriesRLCLoadLib/Series RLC Load  Commented=on  LConnTagsString=a  RConnTagsString=__new0  NominalVoltage=230  NominalFrequency=50  ActivePower=16387.5  InductivePower=5386.311  CapacitivePower=0  Setx0=off  InitialVoltage=0  SetiL0=off  InitialCurrent=0  Measurements=None  LoadType=constant Z
  Series RLC Load28 : spsSeriesRLCLoadLib/Series RLC Load  Commented=on  LConnTagsString=a  RConnTagsString=__new0  NominalVoltage=230  NominalFrequency=50  ActivePower=5462.5  InductivePower=1795.437  CapacitivePower=0  Setx0=off  InitialVoltage=0  SetiL0=off  InitialCurrent=0  Measurements=None  LoadType=constant Z
  Series RLC Load29 : spsSeriesRLCLoadLib/Series RLC Load  Commented=on  LConnTagsString=a  RConnTagsString=__new0  NominalVoltage=230  NominalFrequency=50  ActivePower=6555  InductivePower=2154.52  CapacitivePower=0  Setx0=off  InitialVoltage=0  SetiL0=off  InitialCurrent=0  Measurements=None  LoadType=constant Z
  Series RLC Load3 : spsSeriesRLCLoadLib/Series RLC Load  Commented=on  LConnTagsString=a  RConnTagsString=__new0  NominalVoltage=230  NominalFrequency=50  ActivePower=29497.5  InductivePower=9695.359  CapacitivePower=0  Setx0=off  InitialVoltage=0  SetiL0=off  InitialCurrent=0  Measurements=None  LoadType=constant Z
  Series RLC Load30 : spsSeriesRLCLoadLib/Series RLC Load  Commented=on  LConnTagsString=a  RConnTagsString=__new0  NominalVoltage=230  NominalFrequency=50  ActivePower=3933  InductivePower=1292.715  CapacitivePower=0  Setx0=off  InitialVoltage=0  SetiL0=off  InitialCurrent=0  Measurements=None  LoadType=constant Z
  Series RLC Load31 : spsSeriesRLCLoadLib/Series RLC Load  Commented=on  LConnTagsString=a  RConnTagsString=__new0  NominalVoltage=230  NominalFrequency=50  ActivePower=19228  InductivePower=6319.938  CapacitivePower=0  Setx0=off  InitialVoltage=0  SetiL0=off  InitialCurrent=0  Measurements=None  LoadType=constant Z
  Series RLC Load32 : spsSeriesRLCLoadLib/Series RLC Load  Commented=on  LConnTagsString=a  RConnTagsString=__new0  NominalVoltage=230  NominalFrequency=50  ActivePower=16169  InductivePower=5314.493  CapacitivePower=0  Setx0=off  InitialVoltage=0  SetiL0=off  InitialCurrent=0  Measurements=None  LoadType=constant Z
  Series RLC Load33 : spsSeriesRLCLoadLib/Series RLC Load  Commented=on  LConnTagsString=a  RConnTagsString=__new0  NominalVoltage=230  NominalFrequency=50  ActivePower=15976.5  InductivePower=4955.406  CapacitivePower=0  Setx0=off  InitialVoltage=0  SetiL0=off  InitialCurrent=0  Measurements=None  LoadType=constant Z
  Series RLC Load4 : spsSeriesRLCLoadLib/Series RLC Load  Commented=on  LConnTagsString=a  RConnTagsString=__new0  NominalVoltage=230  NominalFrequency=50  ActivePower=17480  InductivePower=5745.398  CapacitivePower=0  Setx0=off  InitialVoltage=0  SetiL0=off  InitialCurrent=0  Measurements=None  LoadType=constant Z
  Series RLC Load40 : spsSeriesRLCLoadLib/Series RLC Load  Commented=on  LConnTagsString=a  RConnTagsString=__new0  NominalVoltage=230  NominalFrequency=50  ActivePower=9832.5  InductivePower=3231.786  CapacitivePower=0  Setx0=off  InitialVoltage=0  SetiL0=off  InitialCurrent=0  Measurements=None  LoadType=constant Z
  Series RLC Load41 : spsSeriesRLCLoadLib/Series RLC Load  Commented=on  LConnTagsString=a  RConnTagsString=__new0  NominalVoltage=230  NominalFrequency=50  ActivePower=9832.5  InductivePower=3231.786  CapacitivePower=0  Setx0=off  InitialVoltage=0  SetiL0=off  InitialCurrent=0  Measurements=None  LoadType=constant Z
  Series RLC Load42 : spsSeriesRLCLoadLib/Series RLC Load  Commented=on  LConnTagsString=a  RConnTagsString=__new0  NominalVoltage=230  NominalFrequency=50  ActivePower=11143.5  InductivePower=3662.691  CapacitivePower=0  Setx0=off  InitialVoltage=0  SetiL0=off  InitialCurrent=0  Measurements=None  LoadType=constant Z
  Series RLC Load{43..48,52..60} (15 alike) : spsSeriesRLCLoadLib/Series RLC Load  Commented=on  LConnTagsString=a  RConnTagsString=__new0  NominalVoltage=230  NominalFrequency=50  ActivePower=9500  InductivePower=3122.5  CapacitivePower=0  Setx0=off  InitialVoltage=0  SetiL0=off  InitialCurrent=0  Measurements=None  LoadType=constant Z
  Series RLC Load5 : spsSeriesRLCLoadLib/Series RLC Load  Commented=on  LConnTagsString=a  RConnTagsString=__new0  NominalVoltage=230  NominalFrequency=50  ActivePower=21850  InductivePower=7181.74  CapacitivePower=0  Setx0=off  InitialVoltage=0  SetiL0=off  InitialCurrent=0  Measurements=None  LoadType=constant Z
  Series RLC Load6 : spsSeriesRLCLoadLib/Series RLC Load  LConnTagsString=a  RConnTagsString=__new0  NominalVoltage=230  NominalFrequency=50  ActivePower=22287  InductivePower=7325.383  CapacitivePower=0  Setx0=off  InitialVoltage=0  SetiL0=off  InitialCurrent=0  Measurements=None  LoadType=constant Z
  Series RLC Load64 : spsSeriesRLCLoadLib/Series RLC Load  Commented=on  LConnTagsString=a  RConnTagsString=__new0  NominalVoltage=230  NominalFrequency=50  ActivePower=5899.5  InductivePower=1939.072  CapacitivePower=0  Setx0=off  InitialVoltage=0  SetiL0=off  InitialCurrent=0  Measurements=None  LoadType=constant Z
  Series RLC Load65 : spsSeriesRLCLoadLib/Series RLC Load  Commented=on  LConnTagsString=a  RConnTagsString=__new0  NominalVoltage=230  NominalFrequency=50  ActivePower=2622  InductivePower=816.8097  CapacitivePower=0  Setx0=off  InitialVoltage=0  SetiL0=off  InitialCurrent=0  Measurements=None  LoadType=constant Z
  Series RLC Load66 : spsSeriesRLCLoadLib/Series RLC Load  Commented=on  LConnTagsString=a  RConnTagsString=__new0  NominalVoltage=230  NominalFrequency=50  ActivePower=3496  InductivePower=1149.08  CapacitivePower=0  Setx0=off  InitialVoltage=0  SetiL0=off  InitialCurrent=0  Measurements=None  LoadType=constant Z
  Series RLC Load67 : spsSeriesRLCLoadLib/Series RLC Load  Commented=on  LConnTagsString=a  RConnTagsString=__new0  NominalVoltage=230  NominalFrequency=50  ActivePower=6118  InductivePower=2010.889  CapacitivePower=0  Setx0=off  InitialVoltage=0  SetiL0=off  InitialCurrent=0  Measurements=None  LoadType=constant Z
  Series RLC Load68 : spsSeriesRLCLoadLib/Series RLC Load  Commented=on  LConnTagsString=a  RConnTagsString=__new0  NominalVoltage=230  NominalFrequency=50  ActivePower=4151.5  InductivePower=1364.532  CapacitivePower=0  Setx0=off  InitialVoltage=0  SetiL0=off  InitialCurrent=0  Measurements=None  LoadType=constant Z
  Series RLC Load69 : spsSeriesRLCLoadLib/Series RLC Load  Commented=on  LConnTagsString=a  RConnTagsString=__new0  NominalVoltage=230  NominalFrequency=50  ActivePower=218.5  InductivePower=71.81  CapacitivePower=0  Setx0=off  InitialVoltage=0  SetiL0=off  InitialCurrent=0  Measurements=None  LoadType=constant Z
  Series RLC Load7 : spsSeriesRLCLoadLib/Series RLC Load  LConnTagsString=a  RConnTagsString=__new0  NominalVoltage=230  NominalFrequency=50  ActivePower=23379.5  InductivePower=7684.47  CapacitivePower=0  Setx0=off  InitialVoltage=0  SetiL0=off  InitialCurrent=0  Measurements=None  LoadType=constant PQ
  Series RLC Load70 : spsSeriesRLCLoadLib/Series RLC Load  Commented=on  LConnTagsString=a  RConnTagsString=__new0  NominalVoltage=230  NominalFrequency=50  ActivePower=13328.5  InductivePower=4380.866  CapacitivePower=0  Setx0=off  InitialVoltage=0  SetiL0=off  InitialCurrent=0  Measurements=None  LoadType=constant Z
  Series RLC Load71 : spsSeriesRLCLoadLib/Series RLC Load  Commented=on  LConnTagsString=a  RConnTagsString=__new0  NominalVoltage=230  NominalFrequency=50  ActivePower=151435  InductivePower=45626.91  CapacitivePower=0  Setx0=off  InitialVoltage=0  SetiL0=off  InitialCurrent=0  Measurements=None  LoadType=constant Z
  Series RLC Load72 : spsSeriesRLCLoadLib/Series RLC Load  Commented=on  LConnTagsString=a  RConnTagsString=__new0  NominalVoltage=230  NominalFrequency=50  ActivePower=10051  InductivePower=3303.604  CapacitivePower=0  Setx0=off  InitialVoltage=1500000  SetiL0=off  InitialCurrent=0  Measurements=None  LoadType=constant Z
  Series RLC Load73 : spsSeriesRLCLoadLib/Series RLC Load  Commented=on  LConnTagsString=a  RConnTagsString=__new0  NominalVoltage=230  NominalFrequency=50  ActivePower=12891.5  InductivePower=4237.231  CapacitivePower=0  Setx0=off  InitialVoltage=0  SetiL0=off  InitialCurrent=0  Measurements=None  LoadType=constant Z
  Series RLC Load74 : spsSeriesRLCLoadLib/Series RLC Load  Commented=on  LConnTagsString=a  RConnTagsString=__new0  NominalVoltage=230  NominalFrequency=50  ActivePower=12017.5  InductivePower=3949.961  CapacitivePower=0  Setx0=off  InitialVoltage=0  SetiL0=off  InitialCurrent=0  Measurements=None  LoadType=constant Z
  Series RLC Load75 : spsSeriesRLCLoadLib/Series RLC Load  Commented=on  LConnTagsString=a  RConnTagsString=__new0  NominalVoltage=230  NominalFrequency=50  ActivePower=9832.5  InductivePower=3231.786  CapacitivePower=0  Setx0=off  InitialVoltage=0  SetiL0=off  InitialCurrent=0  Measurements=None  LoadType=constant Z
  Series RLC Load76 : spsSeriesRLCLoadLib/Series RLC Load  Commented=on  LConnTagsString=a  RConnTagsString=__new0  NominalVoltage=230  NominalFrequency=50  ActivePower=15732  InductivePower=5170.858  CapacitivePower=0  Setx0=off  InitialVoltage=0  SetiL0=off  InitialCurrent=0  Measurements=None  LoadType=constant Z
  Series RLC Load77 : spsSeriesRLCLoadLib/Series RLC Load  Commented=on  LConnTagsString=a  RConnTagsString=__new0  NominalVoltage=230  NominalFrequency=50  ActivePower=13110  InductivePower=4309.049  CapacitivePower=0  Setx0=off  InitialVoltage=0  SetiL0=off  InitialCurrent=0  Measurements=None  LoadType=constant Z
  Series RLC Load78 : spsSeriesRLCLoadLib/Series RLC Load  Commented=on  LConnTagsString=a  RConnTagsString=__new0  NominalVoltage=230  NominalFrequency=50  ActivePower=17840  InductivePower=5745.398  CapacitivePower=0  Setx0=off  InitialVoltage=0  SetiL0=off  InitialCurrent=0  Measurements=None  LoadType=constant Z
  Series RLC Load8 : spsSeriesRLCLoadLib/Series RLC Load  LConnTagsString=a  RConnTagsString=__new0  NominalVoltage=230  NominalFrequency=50  ActivePower=18572.5  InductivePower=6104.48  CapacitivePower=0  Setx0=off  InitialVoltage=0  SetiL0=off  InitialCurrent=0  Measurements=None  LoadType=constant PQ
  Three-Phase PI Section Line : spsThreePhasePISectionLineLib/Three-Phase PI Section Line  Commented=on  LConnTagsString=a|b|c  RConnTagsString=A|B|C  Length=0.225  Frequency=50  Resistances=[ 0.01273 0.3864]  Inductances="[ 0.9337e-3  4.1264e-3]"  Capacitances=[12.74e-9 7.751e-9]
  Three-Phase PI Section Line1 : spsThreePhasePISectionLineLib/Three-Phase PI Section Line  LConnTagsString=a|b|c  RConnTagsString=A|B|C  Length=0.25  Frequency=50  Resistances=[ 0.01273 0.3864]  Inductances="[ 0.9337e-3  4.1264e-3]"  Capacitances=[12.74e-9 7.751e-9]
  Three-Phase PI Section Line{5,7..18} (13 alike) : spsThreePhasePISectionLineLib/Three-Phase PI Section Line  Commented=on  LConnTagsString=a|b|c  RConnTagsString=A|B|C  Length=0.3  Frequency=50  Resistances=[ 0.01273 0.3864]  Inductances="[ 0.9337e-3  4.1264e-3]"  Capacitances=[12.74e-9 7.751e-9]
  Three-Phase PI Section Line2 : spsThreePhasePISectionLineLib/Three-Phase PI Section Line  LConnTagsString=a|b|c  RConnTagsString=A|B|C  Length=0.3  Frequency=50  Resistances=[ 0.01273 0.3864]  Inductances="[ 0.9337e-3  4.1264e-3]"  Capacitances=[12.74e-9 7.751e-9]
  Three-Phase PI Section Line3 : spsThreePhasePISectionLineLib/Three-Phase PI Section Line  LConnTagsString=a|b|c  RConnTagsString=A|B|C  Length=0.3  Frequency=50  Resistances=[ 0.01273 0.3864]  Inductances="[ 0.9337e-3  4.1264e-3]"  Capacitances=[12.74e-9 7.751e-9]
  Three-Phase PI Section Line4 : spsThreePhasePISectionLineLib/Three-Phase PI Section Line  LConnTagsString=a|b|c  RConnTagsString=A|B|C  Length=0.3  Frequency=50  Resistances=[ 0.01273 0.3864]  Inductances="[ 0.9337e-3  4.1264e-3]"  Capacitances=[12.74e-9 7.751e-9]
  Three-Phase Series RLC Branch : spsThreePhaseSeriesRLCBranchLib/Three-Phase Series RLC Branch  LConnTagsString=A|B|C  RConnTagsString=A|B|C  BranchType=RL  Resistance=1  Inductance=1e-3  Capacitance=1e-6  Measurements=None
  Three-Phase Series RLC Branch1 : spsThreePhaseSeriesRLCBranchLib/Three-Phase Series RLC Branch  LConnTagsString=A|B|C  RConnTagsString=A|B|C  BranchType=L  Resistance=1  Inductance=4e-3  Capacitance=1e-6  Measurements=None
  Three-Phase Transformer (Two Windings){9..10,12,16} (4 alike) : spsThreePhaseTransformerTwoWindingsLib/Three-Phase Transformer (Two Windings)  Commented=on  Winding1Connection=Delta (D11)  Winding2Connection=Yn  CoreType=Three single-phase transformers  SetSaturation=off  Hysteresis=off  DataFile='hysteresis'  SetInitialFlux=off  Measurements=None  UNITS=pu  NominalPower=[ 200000 , 50 ]  Winding1=[ 11e3 , 0.002 , 0.08 ]  Winding2=[ 0.23e3 , 0.002 , 0.08 ]  Rm=500  Lm=500  L0=0.5  Saturation=[ 0,0 ; 0.0024,1.2 ; 1.0,1.52 ]  InitialFluxes=[ 0.8 , -0.8 , 0.7 ]  BreakLoop=off  DiscreteSolver=Trapezoidal iterative  DataType=off  TransfoNumber=1
  Voltage Measurement : spsVoltageMeasurementLib/Voltage Measurement  Commented=on  PhasorSimulation=off  OutputType=Magnitude  PSBequivalent=0
  Voltage Measurement1 : spsVoltageMeasurementLib/Voltage Measurement  Commented=on  PhasorSimulation=off  OutputType=Magnitude  PSBequivalent=0
  Voltage Measurement4 : spsVoltageMeasurementLib/Voltage Measurement  Commented=on  PhasorSimulation=off  OutputType=Complex  PSBequivalent=0
  _ : spsThreePhaseTransformerTwoWindingsLib/Three-Phase Transformer (Two Windings)  Winding1Connection=Delta (D11)  Winding2Connection=Yn  CoreType=Three single-phase transformers  SetSaturation=off  Hysteresis=off  DataFile='hysteresis'  SetInitialFlux=off  Measurements=None  UNITS=pu  NominalPower=[ 100000 , 50 ]  Winding1=[11e3 , 0.002 , 0.08 ]  Winding2=[ 0.23e3 , 0.002 , 0.08 ]  Rm=500  Lm=500  L0=0.5  Saturation=[ 0,0 ; 0.0024,1.2 ; 1.0,1.52 ]  InitialFluxes=[ 0.8 , -0.8 , 0.7 ]  BreakLoop=off  DiscreteSolver=Trapezoidal iterative  DataType=off  TransfoNumber=1
  __ : spsThreePhaseTransformerTwoWindingsLib/Three-Phase Transformer (Two Windings)  Winding1Connection=Delta (D11)  Winding2Connection=Yn  CoreType=Three single-phase transformers  SetSaturation=off  Hysteresis=off  DataFile='hysteresis'  SetInitialFlux=off  Measurements=None  UNITS=pu  NominalPower=[ 300000 , 50 ]  Winding1=[11e3 , 0.002 , 0.08 ]  Winding2=[ 0.23e3 , 0.002 , 0.08 ]  Rm=500  Lm=500  L0=0.5  Saturation=[ 0,0 ; 0.0024,1.2 ; 1.0,1.52 ]  InitialFluxes=[ 0.8 , -0.8 , 0.7 ]  BreakLoop=off  DiscreteSolver=Trapezoidal iterative  DataType=off  TransfoNumber=1
  powergui : spspowerguiLib/powergui  Priority=1  SimulationMode=Discrete  SampleTime=50e-6  frequency=50  Iterations=50  frequencyindice=50  Pbase=100e6  ErrMax=1e-4  UnitsV=kV  UnitsW=MW  buscounter=43  FunctionMessages=off  echomessages=off  EnableUseOfTLC=off  CurrentSourceSwitches=off  DisableSnubberDevices=off  DisableRonSwitches=off  DisableVfSwitches=off  DisplayEquations=off  AutomaticDiscreteSolvers=off  SolverType=Tustin/Backward Euler (TBE)  Interpol=off  ExternalGateDelay=off  methode=off  Ts=100  x0status=blocks  SPID=on  SwTol=0  HookPort=off  NonlinearTolerance=1e-4  nMaxIteration=100  ContinueOnMaxIteration=off  RestoreLinks=warning  ResistiveCurrentMeasurement=off  Frange=[0:2:500]  Ylog=off  Xlog=on  ShowGrid=off  save=off  variable=ZData  structure=0  ZoomFFT=off  StartTime=0.0  cycles=1  DisplayStyle=1  fundamental=60  FreqAxis=off  MaxFrequency=1000  frequencyindicesteady=1  RmsSteady=1  display=off
  thapathali switching : spsThreePhaseSourceLib/Three-Phase Source  InternalConnection=Yg  VoltagePhases=off  Voltage=(11000)*1.00021  PhaseAngle=0.019125  Voltage_phases=[11e3 11e3 11e3]/sqrt(3)  PhaseAngles_phases=[0 -120 +120]  Frequency=50  NonIdealSource=on  SpecifyImpedance=off  Resistance=0.8929  Inductance=16.58e-3  ShortCircuitLevel=100e6  BaseVoltage=11e3  XRratio=7  BusType=swing  Pref=10000  Qref=0  Prefabc=[10e3, 10e3, 10e3]  Qrefabc=[0, 0, 0]  Qmin=-Inf  Qmax=Inf
  wires:
  Voltage Measurement/1 -> RMS1/1
  RMS2/1 -> Display2/1
  Voltage Measurement1/1 -> RMS3/1
  Current Measurement/1 -> RMS/1
  Current Measurement4/1 -> RMS4/1
  RMS1/1 -> Display1/1
  Current Measurement3/1 -> RMS5/1
  RMS5/1 -> Display5/1
  RMS/1 -> Display/1
  RMS4/1 -> Display4/1
  RMS3/1 -> Display3/1
  Voltage Measurement4/1 -> RMS2/1
  1/1 -> RMS6/1
  RMS6/1 -> Display6/1
  0/1 -> RMS7/1
  RMS7/1 -> Display7/1
  connections:
  Bakhundol Kutumba Hotel 200KVA/RConn4 -- Series RLC Load30/LConn1 -- Series RLC Load29/LConn1 -- Series RLC Load28/LConn1
  Three-Phase Transformer (Two Windings)12/LConn1 -- Three-Phase PI Section Line5/RConn1 -- Sajha 500KVA/LConn1 -- Bus*35*/LConn1 -- Three-Phase PI Section Line14/LConn1 -- Three-Phase PI Section Line13/RConn1
  Three-Phase PI Section Line3/RConn3 -- Three-Phase PI Section Line4/LConn3 -- Salik Chwok 200KVA/LConn3
  Three-Phase Transformer (Two Windings)16/RConn4 -- Series RLC Load72/RConn1 -- Series RLC Load70/RConn1 -- Series RLC Load71/RConn1 -- Voltage Measurement4/LConn2 -- Voltage Measurement1/LConn2 -- Voltage Measurement/LConn2
  High Court 200KVA/LConn3 -- Three-Phase PI Section Line11/LConn3 -- Three-Phase Transformer (Two Windings)16/LConn3 -- Three-Phase PI Section Line12/LConn3 -- Three-Phase PI Section Line10/RConn3
  Kandebata Sthan 300KVA/LConn1 -- Bus*30*/LConn1 -- Three-Phase PI Section Line/RConn1 -- Three-Phase Series RLC Branch/LConn1 -- Three-Phase PI Section Line1/LConn1
  Pulchwok Campus Wall 200KVA/LConn2 -- Three-Phase PI Section Line4/RConn2
  Bima Samiti 200KVA/LConn2 -- Three-Phase PI Section Line17/LConn2 -- Sarbanga Hospital 200KVA/LConn2
  Series RLC Load71/LConn1 -- Current Measurement4/RConn1 -- Voltage Measurement1/LConn1
  Three-Phase PI Section Line1/RConn1 -- _/LConn1 -- Bus*41*/LConn1 -- Three-Phase PI Section Line2/LConn1
  Three-Phase PI Section Line7/RConn2 -- Three-Phase PI Section Line5/LConn2 -- .../LConn2 -- Three-Phase PI Section Line10/LConn2 -- Three-Phase PI Section Line18/LConn2 -- Bakhundol Mode 300KVA/LConn2
  Three-Phase PI Section Line9/LConn1 -- Three-Phase PI Section Line8/RConn1 -- Bakhundol Kutumba Hotel 200KVA/LConn1 -- Bus*29*/LConn1
  Three-Phase Transformer (Two Windings)10/LConn3 -- Three-Phase PI Section Line15/RConn3 -- Three-Phase PI Section Line16/LConn3
  Three-Phase PI Section Line5/RConn3 -- Sajha 500KVA/LConn3 -- Three-Phase Transformer (Two Windings)12/LConn3 -- Three-Phase PI Section Line13/RConn3 -- Three-Phase PI Section Line14/LConn3
  Three-Phase PI Section Line8/LConn3 -- Bakhundol Carwash 200KVA/LConn3 -- Three-Phase PI Section Line18/RConn3
  Three-Phase Transformer (Two Windings)10/LConn2 -- Three-Phase PI Section Line15/RConn2 -- Three-Phase PI Section Line16/LConn2
  Three-Phase PI Section Line11/LConn2 -- High Court 200KVA/LConn2 -- Three-Phase Transformer (Two Windings)16/LConn2 -- Three-Phase PI Section Line12/LConn2 -- Three-Phase PI Section Line10/RConn2
  Three-Phase PI Section Line14/LConn2 -- Three-Phase Transformer (Two Windings)12/LConn2 -- Three-Phase PI Section Line13/RConn2 -- Sajha 500KVA/LConn2 -- Three-Phase PI Section Line5/RConn2
  .../LConn3 -- Three-Phase PI Section Line18/LConn3 -- Bakhundol Mode 300KVA/LConn3 -- Three-Phase PI Section Line7/RConn3 -- Three-Phase PI Section Line10/LConn3 -- Three-Phase PI Section Line5/LConn3
  Three-Phase PI Section Line8/LConn1 -- Three-Phase PI Section Line18/RConn1 -- Bakhundol Carwash 200KVA/LConn1 -- Bus*27*/LConn1
  Three-Phase PI Section Line8/RConn3 -- Three-Phase PI Section Line9/LConn3 -- Bakhundol Kutumba Hotel 200KVA/LConn3
  Three-Phase PI Section Line14/RConn2 -- Three-Phase Transformer (Two Windings)9/LConn2 -- Three-Phase PI Section Line15/LConn2
  Series RLC Load46/LConn1 -- Three-Phase Transformer (Two Windings)12/RConn4 -- Series RLC Load48/LConn1 -- Series RLC Load47/LConn1
  Three-Phase PI Section Line7/RConn1 -- Three-Phase PI Section Line18/LConn1 -- Bakhundol Mode 300KVA/LConn1 -- Bus*25*/LConn1
  _/LConn2 -- Three-Phase PI Section Line2/LConn2 -- Three-Phase PI Section Line1/RConn2
  Three-Phase PI Section Line11/LConn1 -- High Court 200KVA/LConn1 -- Bus*37*/LConn1 -- Three-Phase PI Section Line10/RConn1 -- Three-Phase Transformer (Two Windings)16/LConn1 -- Three-Phase PI Section Line12/LConn1
  Three-Phase PI Section Line2/RConn3 -- Three-Phase PI Section Line3/LConn3 -- __/LConn3
  Three-Phase PI Section Line2/RConn1 -- Three-Phase PI Section Line3/LConn1 -- __/LConn1 -- Bus*43*/LConn1
  Three-Phase PI Section Line1/LConn3 -- Kandebata Sthan 300KVA/LConn3 -- Three-Phase PI Section Line/RConn3 -- Three-Phase Series RLC Branch/LConn3
  Bakhundol Carwash 200KVA/LConn2 -- Three-Phase PI Section Line18/RConn2 -- Three-Phase PI Section Line8/LConn2
  _/LConn3 -- Three-Phase PI Section Line2/LConn3 -- Three-Phase PI Section Line1/RConn3
  Series RLC Load33/LConn1 -- Sarwanga Hospital 300KVA/RConn4 -- Series RLC Load32/LConn1 -- Series RLC Load31/LConn1
  Series RLC Load70/LConn1 -- Current Measurement3/RConn1 -- Voltage Measurement/LConn1
  Series RLC Load74/RConn1 -- Jall Utpanna Office 100KVA/RConn4 -- Series RLC Load75/RConn1 -- Series RLC Load73/RConn1
  Series RLC Load6/RConn1 -- Ground/LConn1 -- Series RLC Load8/RConn1 -- Series RLC Load7/RConn1
  Three-Phase PI Section Line4/RConn1 -- Pulchwok Campus Wall 200KVA/LConn1 -- Bus*26*/LConn1
  Series RLC Load52/RConn1 -- Series RLC Load53/RConn1 -- Series RLC Load54/RConn1 -- ../RConn4
  Bima Samiti 200KVA/RConn4 -- Series RLC Load42/LConn1 -- Series RLC Load40/LConn1 -- Series RLC Load41/LConn1
  Series RLC Load43/RConn1 -- Series RLC Load45/RConn1 -- NEA Charging Station/RConn4 -- Series RLC Load44/RConn1
  Three-Phase PI Section Line5/LConn1 -- Three-Phase PI Section Line10/LConn1 -- .../LConn1 -- Bus*24*/LConn1
  Series RLC Load58/RConn1 -- Series RLC Load60/RConn1 -- Three-Phase Transformer (Two Windings)9/RConn4 -- Series RLC Load59/RConn1
  Three-Phase PI Section Line3/RConn2 -- Three-Phase PI Section Line4/LConn2 -- Salik Chwok 200KVA/LConn2
  Bima Samiti 200KVA/LConn3 -- Three-Phase PI Section Line17/LConn3 -- Sarbanga Hospital 200KVA/LConn3
  Bakhundol Carwash 200KVA/RConn4 -- Series RLC Load25/LConn1 -- Series RLC Load26/LConn1 -- Series RLC Load27/LConn1
  .../RConn4 -- Series RLC Load5/RConn1 -- Series RLC Load3/RConn1 -- Series RLC Load4/RConn1
  Three-Phase PI Section Line16/LConn1 -- Three-Phase PI Section Line15/RConn1 -- Three-Phase Transformer (Two Windings)10/LConn1 -- Bus*33*/LConn1
  Bakhundol Mode 300KVA/RConn4 -- Series RLC Load22/LConn1 -- Series RLC Load23/LConn1 -- Series RLC Load24/LConn1
  Series RLC Load68/LConn1 -- Series RLC Load69/LConn1 -- Series RLC Load67/LConn1 -- Pariwar Niyojan 100KVA/RConn4
  Series RLC Load55/RConn1 -- Series RLC Load57/RConn1 -- Three-Phase Transformer (Two Windings)10/RConn4 -- Series RLC Load56/RConn1
  Kandebata Sthan 300KVA/LConn2 -- Three-Phase PI Section Line/RConn2 -- Three-Phase Series RLC Branch/LConn2 -- Three-Phase PI Section Line1/LConn2
  Sarbanga Hospital 200KVA/RConn4 -- Series RLC Load77/LConn1 -- Series RLC Load78/LConn1 -- Series RLC Load76/LConn1
  Voltage Measurement4/LConn1 -- Series RLC Load72/LConn1 -- Current Measurement/RConn1
  Three-Phase PI Section Line2/RConn2 -- Three-Phase PI Section Line3/LConn2 -- __/LConn2
  High Court 200KVA/RConn4 -- Series RLC Load66/LConn1 -- Series RLC Load64/LConn1 -- Series RLC Load65/LConn1
  Three-Phase PI Section Line4/RConn3 -- Pulchwok Campus Wall 200KVA/LConn3
  Three-Phase PI Section Line14/RConn3 -- Three-Phase Transformer (Two Windings)9/LConn3 -- Three-Phase PI Section Line15/LConn3
  Three-Phase PI Section Line8/RConn2 -- Bakhundol Kutumba Hotel 200KVA/LConn2 -- Three-Phase PI Section Line9/LConn2
  Three-Phase PI Section Line3/RConn1 -- Three-Phase PI Section Line4/LConn1 -- Salik Chwok 200KVA/LConn1 -- Bus*23*/LConn1
  Sarbanga Hospital 200KVA/LConn1 -- Three-Phase PI Section Line17/LConn1 -- Bima Samiti 200KVA/LConn1 -- Bus*22*/LConn1
  Three-Phase PI Section Line14/RConn1 -- Three-Phase Transformer (Two Windings)9/LConn1 -- Bus*39*/LConn1 -- Three-Phase PI Section Line15/LConn1
  Current Measurement4/LConn1 -- Three-Phase Transformer (Two Windings)16/RConn3
  Current Measurement3/LConn1 -- Three-Phase Transformer (Two Windings)16/RConn2
  Three-Phase PI Section Line9/RConn2 -- Sarwanga Hospital 300KVA/LConn2
  Three-Phase Transformer (Two Windings)12/RConn1 -- Series RLC Load48/RConn1 -- Bus*34*/LConn1
  Three-Phase PI Section Line11/RConn2 -- Pariwar Niyojan 100KVA/LConn2
  Series RLC Load52/LConn1 -- ../RConn1 -- Bus*12*/LConn1
  Bima Samiti 200KVA/RConn3 -- Series RLC Load42/RConn1
  ../RConn3 -- Series RLC Load54/LConn1
  Jall Utpanna Office 100KVA/RConn3 -- Series RLC Load74/LConn1
  Three-Phase Transformer (Two Windings)10/RConn3 -- Series RLC Load57/LConn1
  Three-Phase PI Section Line9/RConn3 -- Sarwanga Hospital 300KVA/LConn3
  Sarwanga Hospital 300KVA/RConn1 -- Series RLC Load31/RConn1 -- Bus*8*/LConn1
  Three-Phase PI Section Line16/RConn2 -- ../LConn2
  Series RLC Load30/RConn1 -- Bakhundol Kutumba Hotel 200KVA/RConn3
  Sarbanga Hospital 200KVA/RConn1 -- Series RLC Load78/RConn1 -- Bus*17*/LConn1
  Three-Phase PI Section Line13/LConn1 -- NEA Charging Station/LConn1 -- Bus*20*/LConn1
  Series RLC Load58/LConn1 -- Three-Phase Transformer (Two Windings)9/RConn1 -- Bus*38*/LConn1
  NEA Charging Station/RConn2 -- Series RLC Load44/LConn1
  Series RLC Load47/RConn1 -- Three-Phase Transformer (Two Windings)12/RConn2
  Series RLC Load22/RConn1 -- Bakhundol Mode 300KVA/RConn1 -- Bus*4*/LConn1
  Series RLC Load76/RConn1 -- Sarbanga Hospital 200KVA/RConn3
  _/RConn3 -- Jwagal Chowk Load/LConn3
  Series RLC Load4/LConn1 -- .../RConn2
  Three-Phase PI Section Line11/RConn1 -- Pariwar Niyojan 100KVA/LConn1 -- Bus*18*/LConn1
  Series RLC Load77/RConn1 -- Sarbanga Hospital 200KVA/RConn2
  Salik Chwok 200KVA/RConn1 -- Salik Chowk Load/LConn1 -- Bus*2*/LConn1
  Series RLC Load64/RConn1 -- High Court 200KVA/RConn2
  Jall Utpanna Office 100KVA/RConn2 -- Series RLC Load73/LConn1
  Three-Phase Transformer (Two Windings)9/RConn2 -- Series RLC Load59/LConn1
  Series RLC Load75/LConn1 -- Jall Utpanna Office 100KVA/RConn1 -- Bus*16*/LConn1
  Three-Phase PI Section Line12/RConn3 -- Jall Utpanna Office 100KVA/LConn3
  Series RLC Load65/RConn1 -- High Court 200KVA/RConn3
  Series RLC Load66/RConn1 -- High Court 200KVA/RConn1 -- Bus*14*/LConn1
  Three-Phase Transformer (Two Windings)9/RConn3 -- Series RLC Load60/LConn1
  Series RLC Load43/LConn1 -- NEA Charging Station/RConn1 -- Bus*11*/LConn1
  Three-Phase PI Section Line12/RConn2 -- Jall Utpanna Office 100KVA/LConn2
  Three-Phase Transformer (Two Windings)10/RConn2 -- Series RLC Load56/LConn1
  Pariwar Niyojan 100KVA/RConn2 -- Series RLC Load67/RConn1
  Three-Phase PI Section Line16/RConn3 -- ../LConn3
  Series RLC Load27/RConn1 -- Bakhundol Carwash 200KVA/RConn3
  Series RLC Load26/RConn1 -- Bakhundol Carwash 200KVA/RConn2
  _/RConn2 -- Jwagal Chowk Load/LConn2
  Series RLC Load5/LConn1 -- .../RConn3
  Bima Samiti 200KVA/RConn2 -- Series RLC Load41/RConn1
  Series RLC Load55/LConn1 -- Three-Phase Transformer (Two Windings)10/RConn1 -- Bus*32*/LConn1
  Pulchwok Campus Wall 200KVA/RConn1 -- Pulchowk Campus Load/LConn1 -- Bus*3*/LConn1
  NEA Charging Station/RConn3 -- Series RLC Load45/LConn1
  Bakhundol Carwash 200KVA/RConn1 -- Series RLC Load25/RConn1 -- Bus*5*/LConn1
  .../RConn1 -- Series RLC Load3/LConn1 -- Bus*7*/LConn1
  Series RLC Load23/RConn1 -- Bakhundol Mode 300KVA/RConn2
  NEA Charging Station/LConn3 -- Three-Phase PI Section Line13/LConn3
  Sarwanga Hospital 300KVA/LConn1 -- Three-Phase PI Section Line9/RConn1 -- Bus*28*/LConn1
  ../RConn2 -- Series RLC Load53/LConn1
  Series RLC Load29/RConn1 -- Bakhundol Kutumba Hotel 200KVA/RConn2
  _/RConn1 -- Jwagal Chowk Load/LConn1 -- Bus*40*/LConn1
  Series RLC Load32/RConn1 -- Sarwanga Hospital 300KVA/RConn2
  Series RLC Load40/RConn1 -- Bima Samiti 200KVA/RConn1 -- Bus*10*/LConn1
  __/RConn1 -- HImalaya Hotel Load/LConn1 -- Bus*42*/LConn1
  Bakhundol Kutumba Hotel 200KVA/RConn1 -- Series RLC Load28/RConn1 -- Bus*6*/LConn1
  Pariwar Niyojan 100KVA/RConn3 -- Series RLC Load68/RConn1
  Series RLC Load46/RConn1 -- Three-Phase Transformer (Two Windings)12/RConn3
  NEA Charging Station/LConn2 -- Three-Phase PI Section Line13/LConn2
  Series RLC Load69/RConn1 -- Pariwar Niyojan 100KVA/RConn1 -- Bus*15*/LConn1
  Kandebata Sthan 300KVA/RConn1 -- Kandevatasthan Load/LConn1 -- Bus*9*/LConn1
  Series RLC Load24/RConn1 -- Bakhundol Mode 300KVA/RConn3
  Jall Utpanna Office 100KVA/LConn1 -- Three-Phase PI Section Line12/RConn1 -- Bus*19*/LConn1
  Current Measurement/LConn1 -- Three-Phase Transformer (Two Windings)16/RConn1 -- Bus*36*/LConn1
  Series RLC Load33/RConn1 -- Sarwanga Hospital 300KVA/RConn3
  Pariwar Niyojan 100KVA/LConn3 -- Three-Phase PI Section Line11/RConn3
  ../LConn1 -- Three-Phase PI Section Line16/RConn1 -- Bus*21*/LConn1
  Sajha 500KVA/RConn1 -- Series RLC Load1/LConn1 -- Bus*1*/LConn1
  Series RLC Load2/LConn1 -- Sajha 500KVA/RConn2
  Series RLC Load21/LConn1 -- Sajha 500KVA/RConn3
  Sajha 500KVA/RConn4 -- Series RLC Load21/RConn1 -- Series RLC Load2/RConn1 -- Series RLC Load1/RConn1
  0/LConn1 -- Three-Phase Series RLC Branch/RConn1
  0/LConn2 -- Three-Phase Series RLC Branch/RConn2
  0/LConn3 -- Three-Phase Series RLC Branch/RConn3
  0/RConn1 -- Three-Phase Series RLC Branch1/LConn1
  0/RConn2 -- Three-Phase Series RLC Branch1/LConn2
  0/RConn3 -- Three-Phase Series RLC Branch1/LConn3
  Three-Phase Series RLC Branch1/RConn1 -- ./LConn1 -- Bus*31*/LConn1
  ./LConn2 -- Three-Phase Series RLC Branch1/RConn2
  ./LConn3 -- Three-Phase Series RLC Branch1/RConn3
  Load Flow Bus1/LConn1 -- Kandevatasthan Opposite Load/LConn1 -- ./RConn1 -- Bus*13*/LConn1
  thapathali switching/RConn1 -- Load Flow Bus/LConn1 -- 1/LConn1
  thapathali switching/RConn2 -- 1/LConn2
  thapathali switching/RConn3 -- 1/LConn3
  1/RConn1 -- Three-Phase PI Section Line/LConn1
  1/RConn2 -- Three-Phase PI Section Line/LConn2
  1/RConn3 -- Three-Phase PI Section Line/LConn3
  Kandevatasthan Opposite Load/LConn2 -- ./RConn2
  Kandevatasthan Opposite Load/LConn3 -- ./RConn3
  Kandebata Sthan 300KVA/RConn2 -- Kandevatasthan Load/LConn2
  Kandebata Sthan 300KVA/RConn3 -- Kandevatasthan Load/LConn3
  Kandebata Sthan 300KVA/RConn4 -- Kandevatasthan Load/RConn1
  Jwagal Chowk Load/RConn1 -- _/RConn4
  HImalaya Hotel Load/LConn2 -- __/RConn2
  __/RConn3 -- HImalaya Hotel Load/LConn3
  __/RConn4 -- HImalaya Hotel Load/RConn1
  Salik Chwok 200KVA/RConn4 -- Salik Chowk Load/RConn1
  Salik Chowk Load/LConn2 -- Salik Chwok 200KVA/RConn2
  Salik Chwok 200KVA/RConn3 -- Salik Chowk Load/LConn3
  Pulchowk Campus Load/LConn2 -- Pulchwok Campus Wall 200KVA/RConn2
  Pulchowk Campus Load/LConn3 -- Pulchwok Campus Wall 200KVA/RConn3
  Pulchowk Campus Load/RConn1 -- Pulchwok Campus Wall 200KVA/RConn4
